simulink model "script12"  (R2018a)
settings: Solver=ode45  StartTime=0.0  StopTime=10.0  RelTol=1e-3
libraries: simulink x1
settings Model: Creator=User  LastModifiedBy=User

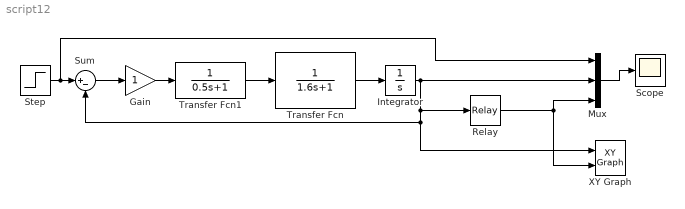
== system script12 ==
  Gain : Gain
  Integrator : Integrator
  Mux : Mux  Inputs=3
  Relay : Relay  OnSwitchValue=1.1  OffSwitchValue=0.95  OnOutputValue=1.5  OffOutputValue=-0.5
  Scope : Scope
  Step : Step  Time=0  SampleTime=0
  Sum : Sum  Inputs=|+-
  Transfer Fcn : TransferFcn  Denominator=[1.6 1]
  Transfer Fcn1 : TransferFcn  Denominator=[0.5 1]
  XY Graph : simulink/Sinks/XY Graph  xmin=0  xmax=2  ymin=-1  ymax=2  st=-1
  wires:
  Step/1 -> Mux/1, Sum/1
  Sum/1 -> Gain/1
  Transfer Fcn1/1 -> Transfer Fcn/1
  Gain/1 -> Transfer Fcn1/1
  Integrator/1 -> Relay/1, XY Graph/1, Sum/2, Mux/2
  Transfer Fcn/1 -> Integrator/1
  Mux/1 -> Scope/1
  Relay/1 -> XY Graph/2, Mux/3
